simulink model "BlockdiagramofSLMPC"  (R2018a)
settings: Solver=VariableStepAuto  StartTime=0.0  StopTime=10.0  RelTol=1e-3
undefined symbols (not defined in the file): A, Aa, B, Ba, C, Ca, Kr, Kx, L
settings Model: Creator=Tarcisio Pinheiro  LastModifiedBy=Tarcisio Pinheiro
settings CodeAppCC: StateflowObjectComments=on

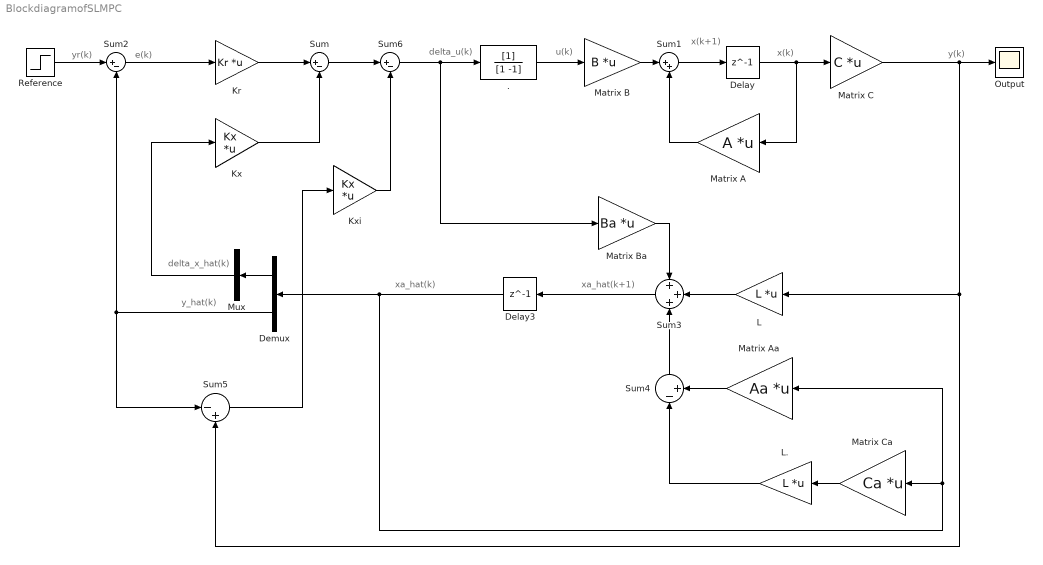
== system BlockdiagramofSLMPC ==
  note: yr(k)
  note: e(k)
  note: delta_u(k)
  note: x(k+1)
  note: x(k)
  note: y(k)
  note: u(k)
  note: xa_hat(k+1)
  note: delta_x_hat(k)
  note: y_hat(k)
  note: xa_hat(k)
  . : DiscreteFilter  Denominator=[1 -1]
  Delay : Delay  DelayLength=1
  Delay3 : Delay  DelayLength=1
  Demux : Demux  Outputs=2
  "Kr " : Gain  Gain=Kr  Multiplication=Matrix(K*u)
  Kx : Gain  Gain=Kx  Multiplication=Matrix(K*u)
  Kxi : Gain  Gain=Kx  Multiplication=Matrix(K*u)
  L : Gain  Gain=L  Multiplication=Matrix(K*u)
  L. : Gain  Gain=L  Multiplication=Matrix(K*u)
  "Matrix A " : Gain  Gain=A  Multiplication=Matrix(K*u)
  Matrix Aa : Gain  Gain=Aa  Multiplication=Matrix(K*u)
  "Matrix B " : Gain  Gain=B  Multiplication=Matrix(K*u)
  Matrix Ba : Gain  Gain=Ba  Multiplication=Matrix(K*u)
  "Matrix C " : Gain  Gain=C  Multiplication=Matrix(K*u)
  Matrix Ca : Gain  Gain=Ca  Multiplication=Matrix(K*u)
  Mux : Mux  Inputs=1
  "Output " : Scope
  Reference : Step  After=3  SampleTime=0
  Sum : Sum  Inputs=|+-
  Sum1 : Sum  Inputs=|++
  Sum2 : Sum  Inputs=|+-
  Sum3 : Sum  Inputs=+++
  Sum4 : Sum  Inputs=|-+
  Sum5 : Sum  Inputs=|-+
  Sum6 : Sum  Inputs=|+-
  wires:
  Reference/1 -> Sum2/1
  "Matrix B "/1 -> Sum1/1
  Delay/1 -> "Matrix A "/1, "Matrix C "/1
  "Matrix C "/1 -> L/1, Sum5/2, "Output "/1
  "Matrix A "/1 -> Sum1/2
  "Kr "/1 -> Sum/1
  Sum1/1 -> Delay/1
  ./1 -> "Matrix B "/1
  L/1 -> Sum3/2
  Sum4/1 -> Sum3/3
  Sum3/1 -> Delay3/1
  Matrix Ca/1 -> L./1
  Matrix Ba/1 -> Sum3/1
  Kx/1 -> Sum/2
  Sum2/1 -> "Kr "/1
  Demux/2 -> Sum5/1, Sum2/2
  Mux/1 -> Kx/1
  Delay3/1 -> Matrix Ca/1, Matrix Aa/1, Demux/1
  Matrix Aa/1 -> Sum4/2
  L./1 -> Sum4/1
  Sum/1 -> Sum6/1
  Sum6/1 -> Matrix Ba/1, ./1
  Sum5/1 -> Kxi/1
  Kxi/1 -> Sum6/2
  Demux/1 -> Mux/1
